simulink library "calculateCXorCZorCM_ul"  (R2020a)
settings: Solver=VariableStepAuto  StartTime=0.0  StopTime=10.0  RelTol=1e-3
undefined symbols (not defined in the file or in its folder): coeffvals
libraries: calcAeroCoeffFromPolynomial_ul x3
settings Model: Creator=Ayaz  LastModifiedBy=Ayaz

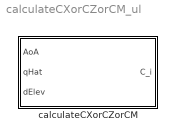
== system calculateCXorCZorCM_ul ==
  calculateCXorCZorCM : Subsystem  mask{C_i_AoA_coeffs=coeffvals, C_i_qHat_coeffs=coeffvals, C_i_dElev_coeffs=coeffvals, C_i_0=1}
      mask prompts: C_i_AoA_coeffs "C_i_AoA polynomial coefficients (c0,c1,c2):"; C_i_qHat_coeffs "C_i_qHat polynomial coefficients (c0,c1,c2):"; C_i_dElev_coeffs "C_i_dElev polynomial coefficients (c0,c1,c2):"; C_i_0 "C_i_0 value"
      mask TypeOptions C_i_AoA_coeffs: C_i_AoA/coeffVals
      mask TypeOptions C_i_qHat_coeffs: C_i_qHat/coeffVals
      mask TypeOptions C_i_dElev_coeffs: C_i_dElev/coeffVals
      mask TypeOptions C_i_0: C_i_0/Value

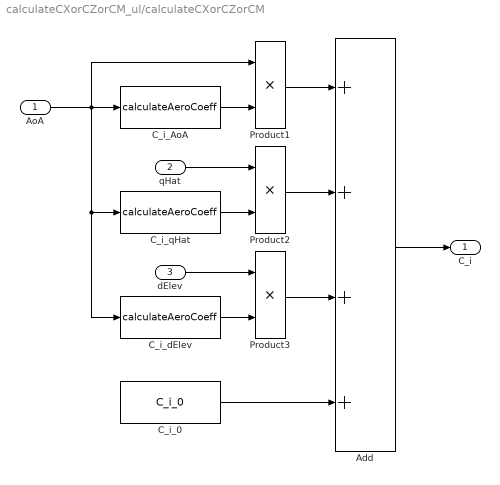
== system calculateCXorCZorCM_ul/calculateCXorCZorCM ==
  AoA : Inport
  qHat : Inport  Port=2
  dElev : Inport  Port=3
  Add : Sum  Inputs=++++
  C_i_0 : Constant  Value=C_i_0
  C_i_AoA : calcAeroCoeffFromPolynomial_ul/calculateAeroCoeff  coeffVals=C_i_AoA_coeffs
  C_i_dElev : calcAeroCoeffFromPolynomial_ul/calculateAeroCoeff  coeffVals=C_i_dElev_coeffs
  C_i_qHat : calcAeroCoeffFromPolynomial_ul/calculateAeroCoeff  coeffVals=C_i_qHat_coeffs
  Product1 : Product
  Product2 : Product
  Product3 : Product
  C_i : Outport
  wires:
  Add/1 -> C_i/1
  AoA/1 -> C_i_dElev/1, C_i_qHat/1, Product1/1, C_i_AoA/1
  C_i_AoA/1 -> Product1/2
  qHat/1 -> Product2/1
  C_i_qHat/1 -> Product2/2
  C_i_dElev/1 -> Product3/2
  dElev/1 -> Product3/1
  C_i_0/1 -> Add/4
  Product3/1 -> Add/3
  Product2/1 -> Add/2
  Product1/1 -> Add/1
